simulink model "Ellipse"  (R2023b)
settings: Solver=FixedStepAuto  StartTime=0.0  StopTime=10.0  RelTol=1e-3
settings Model: Creator=Eric  LastModifiedBy=no
settings SolverCC: AlgebraicLoopSolver=LineSearch
settings DataIOCC: SaveOutput=off  ReturnWorkspaceOutputs=off
settings OptimizationCC: DefaultParameterBehavior=Inlined
settings DebuggingCC: UnconnectedInputMsg=warning  UnconnectedOutputMsg=warning  UnconnectedLineMsg=warning  ArithmeticOperatorsInVariantConditions=warning
settings ModelReferenceCC: EnableRefExpFcnMdlSchedulingChecks=on
settings SFSimCC: SimUseLocalCustomCode=off  CustomCodeUndefinedFunction=UseInterfaceOnly
settings RTWCC: Description=INTECRIO Real-Time Target  SystemTargetFile=irt.tlc  TemplateMakefile=irt_default_tmf  RTWUseLocalCustomCode=off
settings STFCustomTargetCC: UtilityFuncGeneration=Shared location  MatFileLogging=on  GRTInterface=on  SystemTargetFile=irt.tlc
settings GRTTargetCC: UtilityFuncGeneration=Shared location  ParMdlRefBuildCompliant=off  CompOptLevelCompliant=off  ConcurrentExecutionCompliant=off  CombineOutputUpdateFcns=off  CPPClassGenCompliant=off  GRTInterface=on  UseToolchainInfoCompliant=off  GenerateASAP2=on

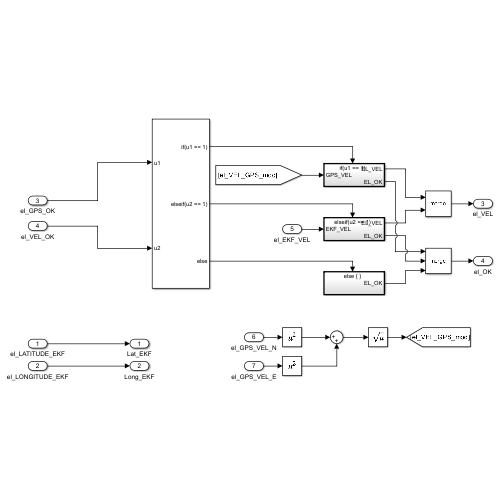
[thumbnail: Simulink's stored preview of the top-level diagram]
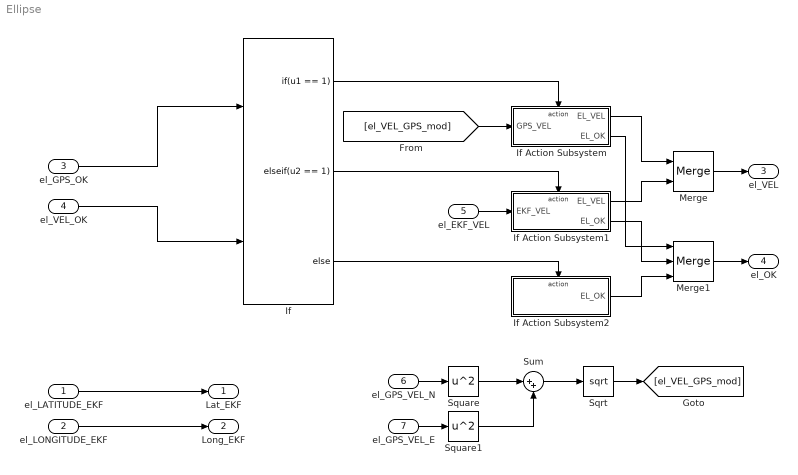
== system Ellipse ==
  el_LATITUDE_EKF : Inport
  el_LONGITUDE_EKF : Inport  Port=2
  el_GPS_OK : Inport  Port=3
  el_VEL_OK : Inport  Port=4
  el_EKF_VEL : Inport  Port=5
  el_GPS_VEL_N : Inport  Port=6
  el_GPS_VEL_E : Inport  Port=7
  If : If  NumInputs=2  IfExpression=u1 == 1  ElseIfExpressions=u2 == 1
  If Action Subsystem : Subsystem  TreatAsAtomicUnit=on
  If Action Subsystem1 : Subsystem  TreatAsAtomicUnit=on
  If Action Subsystem2 : Subsystem  TreatAsAtomicUnit=on
  Merge : Merge
  Merge1 : Merge  Inputs=3
  Sqrt : Sqrt
  Square : Math  Operator=square
  Square1 : Math  Operator=square
  Sum : Sum  Inputs=|++
  Lat_EKF : Outport  VectorParamsAs1DForOutWhenUnconnected=off
  Long_EKF : Outport  Port=2  VectorParamsAs1DForOutWhenUnconnected=off
  el_VEL : Outport  Port=3
  el_OK : Outport  Port=4
  wires:
  el_LONGITUDE_EKF/1 -> Long_EKF/1
  el_LATITUDE_EKF/1 -> Lat_EKF/1
  el_GPS_OK/1 -> If/1
  el_VEL_OK/1 -> If/2
  If/1 -> If Action Subsystem/Action
  [el_VEL_GPS_mod] -> If Action Subsystem/1(GPS_VEL)
  If/2 -> If Action Subsystem1/Action
  el_EKF_VEL/1 -> If Action Subsystem1/1(EKF_VEL)
  If Action Subsystem/1(EL_VEL) -> Merge/1
  If Action Subsystem1/1(EL_VEL) -> Merge/2
  el_GPS_VEL_N/1 -> Square/1
  el_GPS_VEL_E/1 -> Square1/1
  Square/1 -> Sum/1
  Square1/1 -> Sum/2
  Sum/1 -> Sqrt/1
  Sqrt/1 -> [el_VEL_GPS_mod]
  Merge/1 -> el_VEL/1
  If/3 -> If Action Subsystem2/Action
  If Action Subsystem/2(EL_OK) -> Merge1/1
  If Action Subsystem1/2(EL_OK) -> Merge1/2
  If Action Subsystem2/1(EL_OK) -> Merge1/3
  Merge1/1 -> el_OK/1

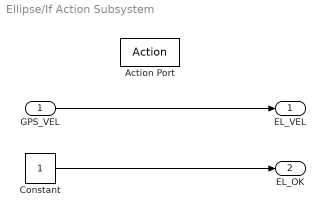
== system Ellipse/If Action Subsystem ==
  GPS_VEL : Inport
  Action Port : ActionPort  ActionPortLabel=if(u1 == 1)
  Constant : Constant
  EL_VEL : Outport
  EL_OK : Outport  Port=2
  wires:
  GPS_VEL/1 -> EL_VEL/1
  Constant/1 -> EL_OK/1

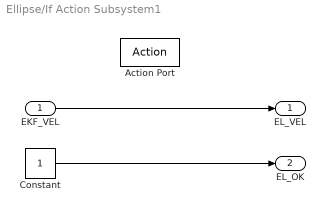
== system Ellipse/If Action Subsystem1 ==
  EKF_VEL : Inport
  Action Port : ActionPort  ActionPortLabel=elseif(u2 == 1)
  Constant : Constant
  EL_VEL : Outport
  EL_OK : Outport  Port=2
  wires:
  EKF_VEL/1 -> EL_VEL/1
  Constant/1 -> EL_OK/1

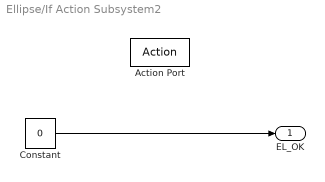
== system Ellipse/If Action Subsystem2 ==
  Action Port : ActionPort  ActionPortLabel=else
  Constant : Constant  Value=0
  EL_OK : Outport
  wires:
  Constant/1 -> EL_OK/1
